simulink model "pendubot_energy_based"  (R2018a)
settings: Solver=ode45  StartTime=0.0  StopTime=20  MaxStep=0.2  RelTol=1e-3
values from neighbouring files (symbols this model uses):
  initialCondition = [q10;q20;qd1_0;qd2_0]    [pendubot_init.m]
  param = [theta1;theta2;theta3;theta4;theta5;g]    [pendubot_init.m]
settings Model: Creator=stefano  LastModifiedBy=Pimentel
settings DataIOCC: ReturnWorkspaceOutputs=on
settings SFSimCC: SimUseLocalCustomCode=on
settings RTWCC: RTWUseLocalCustomCode=on

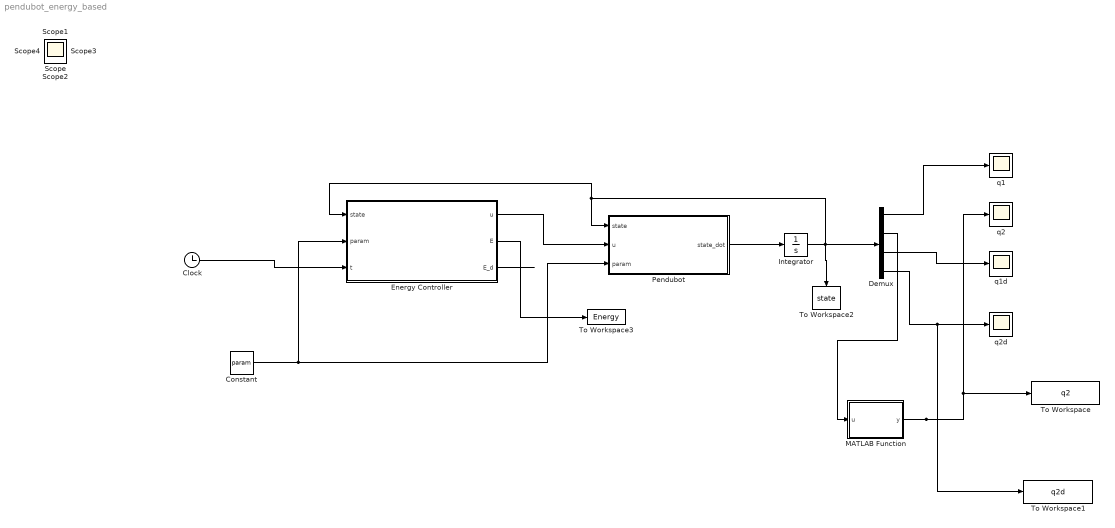
== system pendubot_energy_based ==
  Clock : Clock
  Constant : Constant  Value=param
  Demux : Demux
  Energy Controller : MATLAB Function  TreatAsAtomicUnit=on
  Integrator : Integrator  InitialCondition=initialCondition
  MATLAB Function : MATLAB Function  TreatAsAtomicUnit=on
  Pendubot : MATLAB Function  TreatAsAtomicUnit=on
  To Workspace : ToWorkspace  VariableName=q2  SaveFormat=Timeseries  SampleTime=-1
  To Workspace1 : ToWorkspace  VariableName=q2d  SaveFormat=Timeseries  SampleTime=-1
  To Workspace2 : ToWorkspace  VariableName=state  SaveFormat=Structure With Time  SampleTime=-1
  To Workspace3 : ToWorkspace  VariableName=Energy  SaveFormat=Structure With Time  SampleTime=-1
  "q1 " : Scope
  q1d : Scope
  q2 : Scope
  q2d : Scope
  Scope{,1..4} (5 alike) : Scope
  wires:
  Pendubot/1(state_dot) -> Integrator/1
  Integrator/1 -> To Workspace2/1, Demux/1, Energy Controller/1(state), Pendubot/1(state)
  Constant/1 -> Pendubot/3(param), Energy Controller/2(param)
  Energy Controller/1(u) -> Pendubot/2(u)
  Demux/3 -> q1d/1
  Demux/4 -> To Workspace1/1, q2d/1
  Demux/2 -> MATLAB Function/1(u)
  MATLAB Function/1(y) -> q2/1, To Workspace/1
  Demux/1 -> "q1 "/1
  Clock/1 -> Energy Controller/3(t)
  Energy Controller/2(E) -> To Workspace3/1
  Energy Controller/3(E_d) -> ?

== matlab function pendubot_energy_based/Energy Controller ==
  data: state input; u output; param input; t input; E output; E_d output
function [u,E,E_d] = Energy_Controller(state,param,t) 

kp = 3.55;
kd = 1;
ke = 1.5;

% m1 = param(1);
% m2 = param(2);
% l1 = param(3);
% l2 = param(4);
% lc_1 = param(5);
% lc_2 = param(6);
% I1 = param(7);
% I2 = param(8);
% g = param(9);

% parameters needed to compute the control

theta1 = param(1); 
theta2 = param(2);
theta3 = param(3);
theta4 = param(4);
theta5 = param(5);
g = param(6);

% for the angles I need to be sure that I am normalizing the angles between
% 0 and 2pi while maintaining the sign 

q1 = state(1);
if q1 >= 0
    q1 = mod(q1,2*pi);
else
    q1 = mod(q1,-2*pi);
end
q2 = state(2);
if q2 >= 0
    q2 = mod(q2,2*pi);
else
    q2 = mod(q2,-2*pi);
end
v1 = state(3);
v2 = state(4);

v = [v1;v2];

% Inertia Matrix of the robot needed to compute the enrgy for the creation
% of the control

d11 = theta1 + theta2 + 2*theta3*cos(q2);
d12 = theta2 + theta3*cos(q2);
d21 = d12;
d22 = theta2;

M = [d11 d12; d21 d22];

Kinetic = 1/2 * v'*M*v;
Potential = theta4*g*sin(q1) + theta5*g*sin(q1+q2);

E = Kinetic + Potential;

% Desired values for state and energy in the up up configuration and error
% definition

q1_d = pi/2;
q1d_d = 0;
E_d = (theta4 + theta5)*g;

q1_e = q1 - q1_d;
q1d_e = q1d_d - v1;
E_e = E - E_d;

% subexpression in the control

F = theta2*theta3*sin(q2)*(v1+v2)^2 + theta3^2*cos(q2)*sin(q2)*v1^2 - theta2*theta4*g*cos(q1) + theta3*theta5*g*cos(q2)*cos(q1+q2);


%Gain Matrix for linear Controller

K = [-50.0719  -49.8364  -10.8067   -7.5569];

u = (-kd*F - (theta1*theta2 - theta3^2*cos(q2)^2)*(v1 + kp*q1_e))/((theta1*theta2 - theta3^2*cos(q2)^2)*ke*E_e + kd*theta2);


if t >= 9.4
    % if switching instant has occured then generates the torque as a
    % linear conroller
    u = -K*[q1 - pi/2;q2;v1;v2];
end

== matlab function pendubot_energy_based/Pendubot ==
  data: state input; u input; state_dot output; param input
function state_dot = Pendubot_Model(state,u,param)

% m1 = param(1);
% m2 = param(2);
% l1 = param(3);
% l2 = param(4);
% lc_1 = param(5);
% lc_2 = param(6);
% I1 = param(7);
% I2 = param(8);
% g = param(9);

theta1 = param(1); 
theta2 = param(2);
theta3 = param(3);
theta4 = param(4);
theta5 = param(5);
g = param(6);

%state

% for the angles I need to be sure that I am normalizing the angles between
% 0 and 2pi while maintaining the sign 
q1 = state(1);
if q1 >= 0
    q1 = mod(q1,2*pi);
else
    q1 = mod(q1,-2*pi);
end
q2 = state(2);
if q2 >= 0
    q2 = mod(q2,2*pi);
else
    q2 = mod(q2,-2*pi);
end
v1 = state(3);
v2 = state(4);

%dynamic elements

d11 = theta1 + theta2 + 2*theta3*cos(q2);
d12 = theta2 + theta3*cos(q2);
d21 = d12;
d22 = theta2;
h1 = theta3*sin(q2)*(-v1*v2 -(v1+v2)*v2);
h2 = theta3*sin(q2)*v1^2;
phi1 = theta4*g*cos(q1) + theta5*g*cos(q1+q2);
phi2 = theta5*g*cos(q1+q2);

% d11 = m1*lc_1^2 + m2*(l1^2 + lc_2^2 + 2*l1*lc_2*cos(q2)) + I1 + I2;
% d22 = m2*lc_2^2 + I2;
% d12 = m2*(lc_2^2 + l1*lc_2*cos(q2)) + I2;
% d21 = m2*(lc_2^2 + l1*lc_2*cos(q2)) + I2;
% h1 = -m2*l1*lc_2*sin(q2)*v2^2 - 2*m2*l1*lc_2*sin(q2)*v2*v1;
% h2 = m2*l1*lc_2*sin(q2)*v1^2;
% phi1 = (m1*lc_1 + m2*l1)*g*cos(q1) + m2*lc_2*g*cos(q1+q2);
% phi2 = m2*lc_2*g*cos(q1+q2);

% Matrix of the euler lagrange equations of the robot dynamic
% M(q)*qdd + C(q,qd) + e(q) = [0;tau]

M = [d11 d12; d21 d22];
C = [h1;h2];
e = [phi1;phi2];

%Model in state space

q1_d = v1;
q2_d = v2;
% to find the accelerations I simply invert the dynamic equation from the
% euler lagrange formalism because simpler than extrapolate the correct
% single definintions
q_dd = inv(M)*([u;0] - C - e);
q1_dd = q_dd(1);
q2_dd = q_dd(2);

state_dot = [q1_d;q2_d;q1_dd;q2_dd];

== matlab function pendubot_energy_based/MATLAB Function ==
  data: u input; y output
function y = fcn(u)

y = mod(u,-2*pi);
